simulink model "irsensordebug"  (R2023b)
settings: Solver=FixedStepAuto  StartTime=0.0  StopTime=inf  RelTol=1e-3  EnableMultiTasking=on
libraries: vexarmcortexlib x1
settings Model: ExtModeTrigDuration=25  Creator=shane  LastModifiedBy=shane
settings OptimizationCC: EnhancedBackFolding=on  PassReuseOutputArgsAs=Individual arguments  ZeroExternalMemoryAtStartup=off  ZeroInternalMemoryAtStartup=off  MaxStackSize=64  OptimizeBlockOrder=speed  DifferentSizesBufferReuse=on  OptimizationCustomize=off  EfficientTunableParamExpr=on
settings DebuggingCC: ParameterTunabilityLossMsg=error
settings HardwareCC: ProdBitPerPointer=32  ProdBitPerSizeT=32  ProdBitPerPtrDiffT=32  ProdLargestAtomicInteger=Long  ProdLargestAtomicFloat=Double  ProdWordSize=32  ProdHWDeviceType=ARM Compatible->ARM Cortex
settings SFSimCC: MATLABDynamicMemAlloc=off
settings RTWCC: Description=Embedded Coder  SystemTargetFile=ert.tlc  HardwareBoard=ARM Cortex-based VEX Microcontroller  TLCOptions="-aInlineSetEventsForThisBaseRateFcn=TLC_FALSE -aSuppressMultiTaskScheduler=TLC_FALSE  -aRateBasedStepFcn=0"  TemplateMakefile=ert_default_tmf  Toolchain=GNU Tools for VEX ARM Cortex
settings CodeAppCC: ForceParamTrailComments=on  IgnoreCustomStorageClasses=off  OperatorAnnotations=on  SimulinkDataObjDesc=on  SFDataObjDesc=on  InsertBlockDesc=on
settings ERTTargetCC: SupportContinuousTime=on  ExtModeTransport=1  ExtModeMexFile=ext_serial_win32_comm

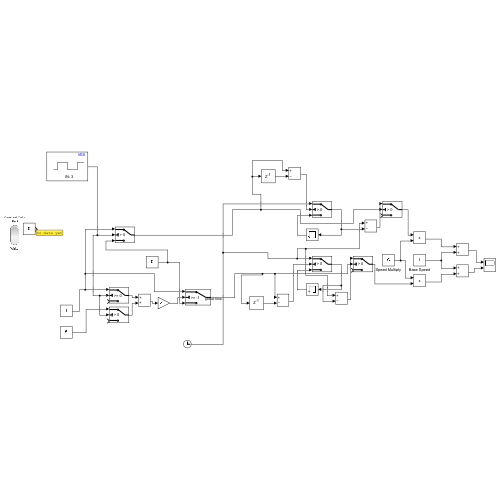
[thumbnail: Simulink's stored preview of the top-level diagram]
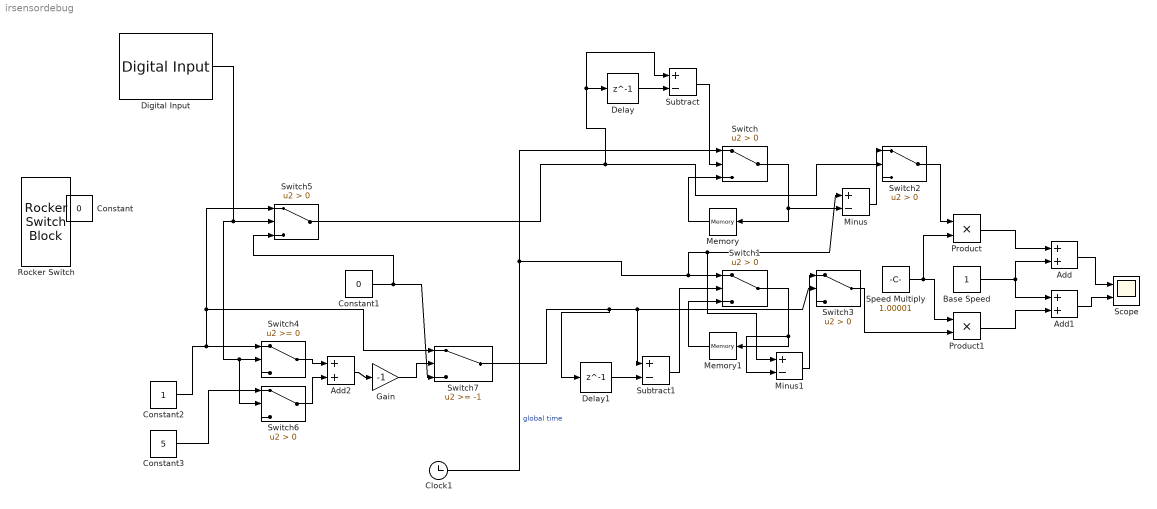
== system irsensordebug ==
  Add : Sum
  Add1 : Sum
  Add2 : Sum
  Base Speed : Constant
  Clock1 : Clock
  Constant : Constant  Value=0
  Constant1 : Constant  Value=0
  Constant2 : Constant
  Constant3 : Constant  Value=5
  Delay : Delay  DelayLength=1  InitialCondition=0
  Delay1 : Delay  DelayLength=1  InitialCondition=0
  Digital Input : vexarmcortexlib/Sensors/Digital Input  inChan=3  SimulationIn=off  SampleTime=0.2
  Gain : Gain  Gain=-1
  Memory : Memory
  Memory1 : Memory
  Minus : Sum  Inputs=+-
  Minus1 : Sum  Inputs=+-
  Product : Product
  Product1 : Product
  Rocker Switch : RockerSwitchBlock
      settings: Values={{'White', 'Black'}, [0 1]}
  Scope : Scope  NumInputPorts=2
  Speed Multiply : Constant  Value=1.00001
  Subtract : Sum  Inputs=+-
  Subtract1 : Sum  Inputs=+-
  Switch{,1..3,5..6} (6 alike) : Switch  Criteria=u2 > Threshold  SaturateOnIntegerOverflow=off  InputSameDT=off
  Switch4 : Switch  SaturateOnIntegerOverflow=off  InputSameDT=off
  Switch7 : Switch  Threshold=-1  SaturateOnIntegerOverflow=off  InputSameDT=off
  wires:
  Clock1/1 -> Minus/1, Minus1/1, Switch1/1, Switch/1  "global time"
  Switch/1 -> Minus/2, Memory/1
  Memory/1 -> Switch/3
  Switch1/1 -> Minus1/2, Memory1/1
  Memory1/1 -> Switch1/3
  Add1/1 -> Scope/2
  Add/1 -> Scope/1
  Product/1 -> Add/1
  Product1/1 -> Add1/2
  Base Speed/1 -> Add/2, Add1/1
  Speed Multiply/1 -> Product/2, Product1/1
  Switch3/1 -> Product1/2
  Switch2/1 -> Product/1
  Digital Input/1 -> Switch6/2, Switch4/2, Switch5/2
  Switch5/1 -> Subtract/1, Delay/1, Switch2/2
  Switch7/1 -> Delay1/1, Subtract1/1, Switch3/2
  Constant3/1 -> Switch6/1
  Constant2/1 -> Switch7/1, Switch5/1, Switch4/1
  Add2/1 -> Gain/1
  Switch4/1 -> Add2/1
  Switch6/1 -> Add2/2
  Gain/1 -> Switch7/2
  Constant1/1 -> Switch7/3, Switch5/3
  Minus/1 -> Switch2/1
  Minus1/1 -> Switch3/1
  Delay/1 -> Subtract/2
  Subtract/1 -> Switch/2
  Delay1/1 -> Subtract1/2
  Subtract1/1 -> Switch1/2
